simulink model "Problem210"  (R2025b)
settings: Solver=VariableStepAuto  StartTime=0.0  StopTime=10.0  RelTol=1e-3
settings Model: Creator=colli  LastModifiedBy=colli

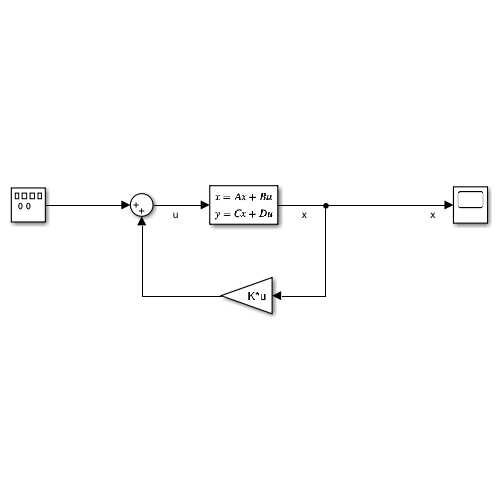
[thumbnail: Simulink's stored preview of the top-level diagram]
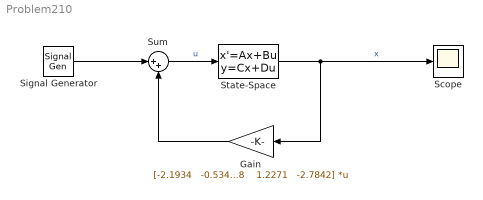
== system Problem210 ==
  Gain : Gain  Gain="[-2.1934   -0.5348    1.2271   -2.7842]"  Multiplication=Matrix(K*u)
  Scope : Scope
      settings: ActiveDisplayYMinimum=-0.21669  ActiveDisplayYMaximum=0.07025
  Signal Generator : SignalGenerator  Units=rad/sec
  State-Space : StateSpace  A=[-9 4 4 -5; 6 -2 -7 9; -5 0 -9 5; 0 -7 0 4]  B=[1; 0; -2; 3]  C=eye(4)  D=[0; 0; 0; 0]  InitialCondition=[1 0 2 0]
  Sum : Sum  Inputs=|++
  wires:
  Signal Generator/1 -> Sum/1
  Sum/1 -> State-Space/1  "u"
  State-Space/1 -> Scope/1, Gain/1  "x"
  Gain/1 -> Sum/2
